simulink model "model_anticipation"  (R2013b)
settings: Solver=ode45  StartTime=0.0  StopTime=10.0  FixedStep=0.2  RelTol=1e-3
undefined symbols (not defined in the file): A, B, C, K, L
settings Model: Creator=Sander  LastModifiedBy=Sander

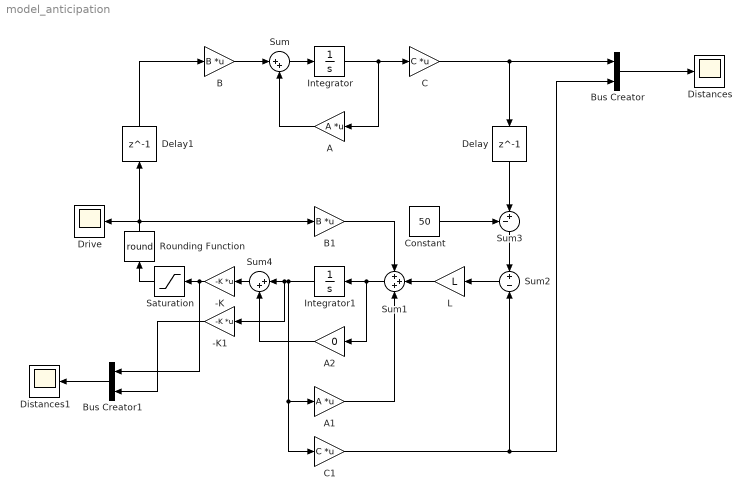
== system model_anticipation ==
  -K : Gain  Gain=-K  Multiplication=Matrix(K*u)
  -K1 : Gain  Gain=-K  Multiplication=Matrix(K*u)
  A : Gain  Gain=A  Multiplication=Matrix(K*u)
  A1 : Gain  Gain=A  Multiplication=Matrix(K*u)
  A2 : Gain  Gain=0
  B : Gain  Gain=B  Multiplication=Matrix(K*u)
  B1 : Gain  Gain=B  Multiplication=Matrix(K*u)
  Bus Creator : BusCreator  Inputs=2
  Bus Creator1 : BusCreator  Inputs=2
  C : Gain  Gain=C  Multiplication=Matrix(K*u)
  C1 : Gain  Gain=C  Multiplication=Matrix(K*u)
  Constant : Constant  Value=50
  Delay : Delay  DelayLength=1  InitialCondition=300  SampleTime=0.05
  Delay1 : Delay  DelayLength=1  InitialCondition=0  SampleTime=0.05
  Distances : Scope
      settings: ShowLegends=on  TimeRange=8.13238770685579  YMin=27.18749999999995  YMax=115.3125
  Distances1 : Scope
      settings: ShowLegends=on  TimeRange=8.13238770685579  YMin=27.18749999999995  YMax=115.3125
  Drive : Scope
      settings: ShowLegends=on  SaveName=ScopeData2
  Integrator : Integrator  InitialCondition=[300;0]
  Integrator1 : Integrator  InitialCondition=[250;0]
  L : Gain  Gain=L
  Rounding Function : Rounding  Operator=round
  Saturation : Saturate  UpperLimit=15  LowerLimit=-15  RndMeth=Round
      settings: LockScale=on
  Sum : Sum  Inputs=|++
  Sum1 : Sum  Inputs=+++
  Sum2 : Sum  Inputs=+|-
  Sum3 : Sum  Inputs=-+|
  Sum4 : Sum  Inputs=|++
  wires:
  A/1 -> Sum/2
  B/1 -> Sum/1
  Sum/1 -> Integrator/1
  Integrator/1 -> C/1, A/1
  Sum1/1 -> A2/1, Integrator1/1
  A1/1 -> Sum1/3
  B1/1 -> Sum1/1
  L/1 -> Sum1/2
  Sum2/1 -> L/1
  Bus Creator/1 -> Distances/1
  C1/1 -> Sum2/2, Bus Creator/2
  C/1 -> Delay/1, Bus Creator/1
  -K/1 -> Bus Creator1/1, Saturation/1
  Sum3/1 -> Sum2/1
  Constant/1 -> Sum3/1
  Rounding Function/1 -> Delay1/1, B1/1, Drive/1
  Saturation/1 -> Rounding Function/1
  Delay/1 -> Sum3/2
  Sum4/1 -> -K/1
  Integrator1/1 -> C1/1, A1/1, -K1/1, Sum4/1
  A2/1 -> Sum4/2
  Bus Creator1/1 -> Distances1/1
  -K1/1 -> Bus Creator1/2
  Delay1/1 -> B/1
